simulink model "pmsm_sysid_fanload"  (R2021a)
settings: Solver=VariableStepAuto  StartTime=0.0  StopTime=29.9  RelTol=1e-3
model workspace (MATLAB code in the model file):
  | np=4; % pole pairs
  | phiv=0.1167; % rotor flux, wb
  | Kt=3/2*np*phiv;
  | f=2e-5; %Nm/(rad/s), resistance air load
  | J=1.74e-2; %kgm*m, inertia
  | L=0.008; %H, inductance
  | Ld=L;
  | Lq=L;
  | Rs=1.74; %Ohm, armature resistance
  | Kp=5; % Prop gain in inner PI
  | Ki=250; % I gain in inner PI
  | Ti = Kp/Ki;
  | h = 1e-1; % Sampling period
  | wN = pi/h; % Nyquist freq
  | wBf = 0.7*wN; % Cutoff freq for AA filter
  | w0f = wBf/2.11; % AA filter param
libraries: simulink x1
settings Model: Creator=kjartan  LastModifiedBy=kjartan
settings SolverCC: AlgebraicLoopSolver=TrustRegion
settings DataIOCC: ReturnWorkspaceOutputs=off
settings DebuggingCC: SFMachineParentedDataDiag=warning  ArithmeticOperatorsInVariantConditions=warning
settings SFSimCC: CustomCodeUndefinedFunction=UseInterfaceOnly

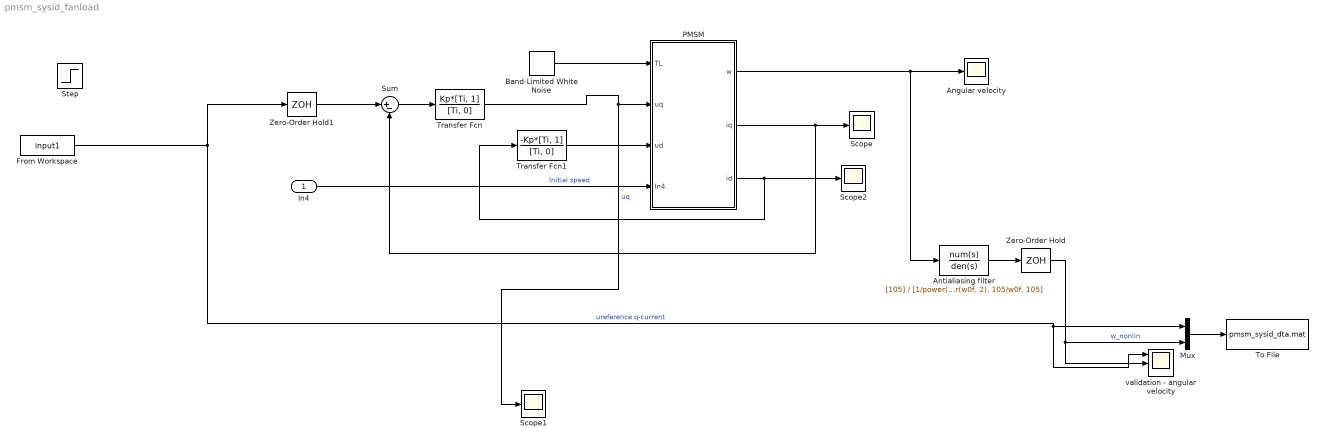
== system pmsm_sysid_fanload ==
  In4 : Inport
  Angular velocity : Scope
  Antialiasing filter : TransferFcn  Numerator=[105]  Denominator=[1/power(w0f,4), 10/power(w0f, 3), 45/power(w0f, 2), 105/w0f, 105]
  Band-Limited White Noise : simulink/Sources/Band-Limited White Noise  Cov=100  Ts=0.1  seed=[23341]
  From Workspace : FromWorkspace  VariableName=input1  SampleTime=h
  Mux : Mux  Inputs=2
  PMSM : Subsystem
  Scope : Scope
  Scope1 : Scope
  Scope2 : Scope
  Step : Step  After=100  SampleTime=0
  Sum : Sum  Inputs=|+-
  To File : ToFile  Filename=pmsm_sysid_dta.mat  MatrixName=uy  SaveFormat=Timeseries
  Transfer Fcn : TransferFcn  Numerator=Kp*[Ti, 1]  Denominator=[Ti, 0]
  Transfer Fcn1 : TransferFcn  Numerator=-Kp*[Ti, 1]  Denominator=[Ti, 0]
  Zero-Order Hold : ZeroOrderHold  SampleTime=h
  Zero-Order Hold1 : ZeroOrderHold  SampleTime=h
  "validation - angular velocity " : Scope  NumInputPorts=3
  wires:
  In4/1 -> PMSM/4(In4)  "Initial speed"
  PMSM/1(w) -> Angular velocity/1, Antialiasing filter/1
  PMSM/2(iq) -> Sum/2, Scope/1
  PMSM/3(id) -> Transfer Fcn1/1, Scope2/1
  Sum/1 -> Transfer Fcn/1
  From Workspace/1 -> Zero-Order Hold1/1, Mux/1, "validation - angular velocity "/1  "ureference q-current"
  Transfer Fcn1/1 -> PMSM/3(ud)
  Zero-Order Hold1/1 -> Sum/1
  Antialiasing filter/1 -> Zero-Order Hold/1
  Zero-Order Hold/1 -> Mux/2, "validation - angular velocity "/2  "w_nonlin"
  Mux/1 -> To File/1
  Transfer Fcn/1 -> Scope1/1, PMSM/2(uq)  "uq"
  Band-Limited White Noise/1 -> PMSM/1(TL)

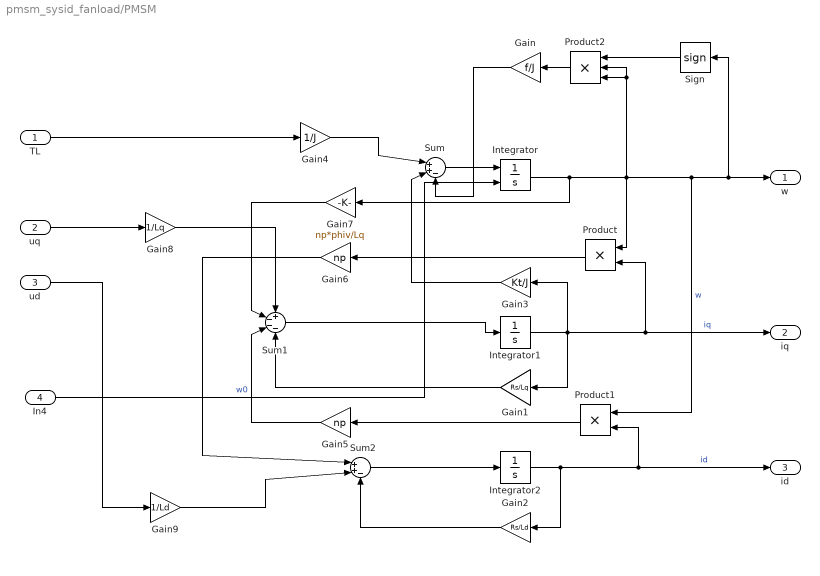
== system pmsm_sysid_fanload/PMSM ==
  TL : Inport
  uq : Inport  Port=2
  ud : Inport  Port=3
  In4 : Inport  Port=4
  Gain : Gain  Gain=f/J
  Gain1 : Gain  Gain=Rs/Lq
  Gain2 : Gain  Gain=Rs/Ld
  Gain3 : Gain  Gain=Kt/J
  Gain4 : Gain  Gain=1/J
  Gain5 : Gain  Gain=np
  Gain6 : Gain  Gain=np
  Gain7 : Gain  Gain=np*phiv/Lq
  Gain8 : Gain  Gain=1/Lq
  Gain9 : Gain  Gain=1/Ld
  Integrator : Integrator  InitialConditionSource=external
  Integrator1 : Integrator
  Integrator2 : Integrator
  Product : Product
  Product1 : Product
  Product2 : Product  Inputs=3
  Sign : Signum
  Sum : Sum  Inputs=|++-
  Sum1 : Sum  Inputs=+---
  Sum2 : Sum  Inputs=|++-
  w : Outport  VectorParamsAs1DForOutWhenUnconnected=off
  iq : Outport  Port=2  VectorParamsAs1DForOutWhenUnconnected=off
  id : Outport  Port=3  VectorParamsAs1DForOutWhenUnconnected=off
  wires:
  Product/1 -> Gain6/1
  Gain9/1 -> Sum2/2
  Gain2/1 -> Sum2/3
  Gain5/1 -> Sum1/3
  Gain/1 -> Sum/3
  Gain8/1 -> Sum1/1
  Product1/1 -> Gain5/1
  Gain3/1 -> Sum/2
  Gain7/1 -> Sum1/2
  In4/1 -> Integrator/2  "w0"
  Integrator1/1 -> Gain3/1, Gain1/1, iq/1, Product/2  "iq"
  uq/1 -> Gain8/1
  Sum1/1 -> Integrator1/1
  Integrator/1 -> Gain7/1, Product2/2, Product2/3, Product/1, Sign/1, w/1, Product1/1  "w"
  Gain6/1 -> Sum2/1
  Sum2/1 -> Integrator2/1
  Gain1/1 -> Sum1/4
  Integrator2/1 -> Gain2/1, id/1, Product1/2  "id"
  ud/1 -> Gain9/1
  Sum/1 -> Integrator/1
  TL/1 -> Gain4/1
  Gain4/1 -> Sum/1
  Product2/1 -> Gain/1
  Sign/1 -> Product2/1
